simulink model "Lab_1_"  (R2022a)
settings: Solver=VariableStepAuto  StartTime=0.0  StopTime=50  RelTol=1e-3
undefined symbols (not defined in the file or in its folder): den, num
settings Model: Creator=pdidd  LastModifiedBy=pdidd

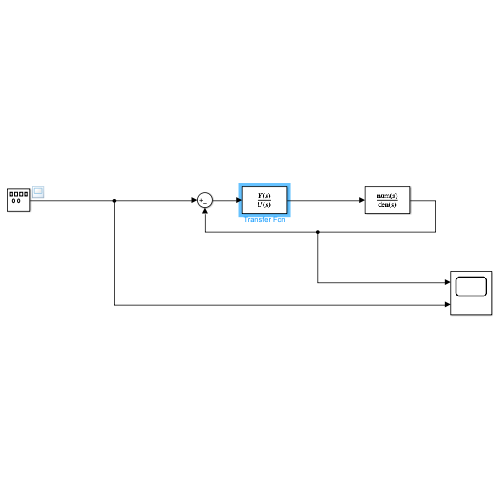
[thumbnail: Simulink's stored preview of the top-level diagram]
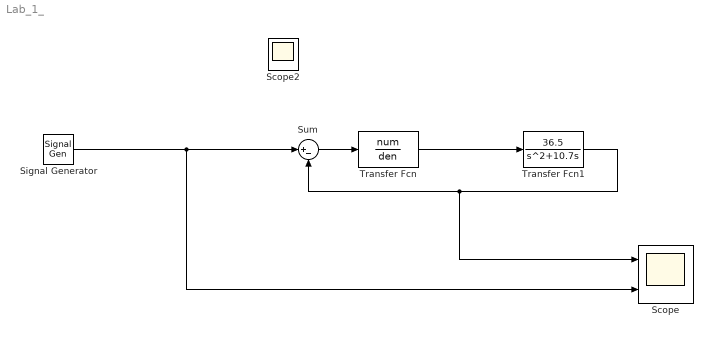
== system Lab_1_ ==
  Scope : Scope  NumInputPorts=2
  Signal Generator : SignalGenerator  WaveForm=square  Amplitude=2.5  Frequency=0.4  Units=rad/sec
  Sum : Sum  Inputs=|+-
  Transfer Fcn : TransferFcn  Numerator=num  Denominator=den
  Transfer Fcn1 : TransferFcn  Numerator=[36.5]  Denominator=[1 10.7 0]
  Scope2 : Scope
  wires:
  Transfer Fcn/1 -> Transfer Fcn1/1
  Transfer Fcn1/1 -> Sum/2, Scope/1
  Sum/1 -> Transfer Fcn/1
  Signal Generator/1 -> Sum/1, Scope/2
